simulink library "INP_IMU"  (R2024b)
settings: Solver=VariableStepAuto  StartTime=0.0  StopTime=10.0  RelTol=1e-3
libraries: INP_IMU_Comp2 x1, INP_IMU_ManOver2 x1, INP_IMU_ManOverAngRat2 x1, INP_IMU_PrepAngRat2 x1, INP_IMU_Prep2 x1
settings Model: Creator=blatak  LastModifiedBy=jmbsp
settings RTWCC: GPUComputeCapability=3.5

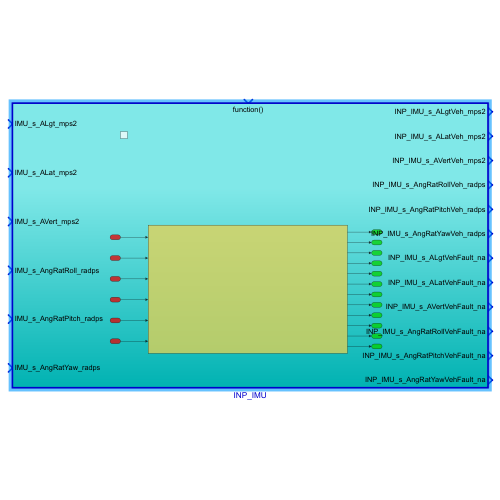
[thumbnail: Simulink's stored preview of the top-level diagram]
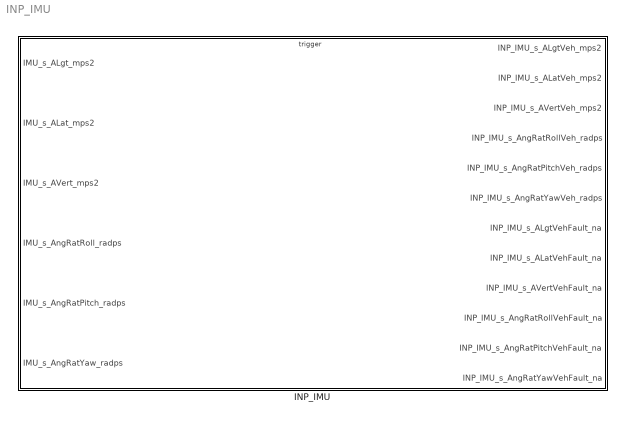
== system INP_IMU ==
  INP_IMU : Subsystem  Description=|  TreatAsAtomicUnit=on
      | Block recalculates the raw acceleration value from sensor position to cog, low
      | pass filtering, manual switches and saturation

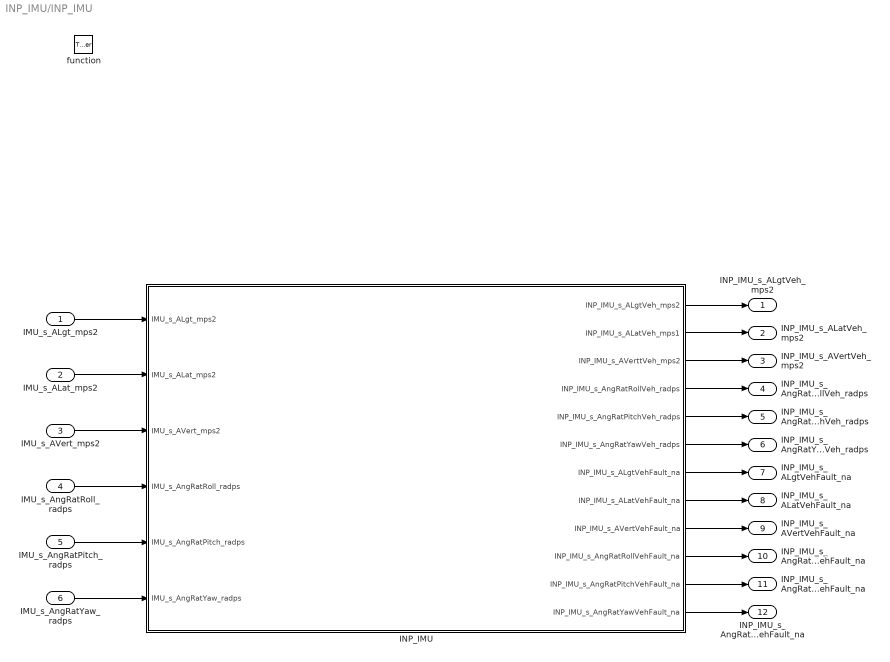
== system INP_IMU/INP_IMU ==
  IMU_s_ALgt_mps2 : Inport  Description=IMU Longitudinal acceleration - raw measured value from sensor
  IMU_s_ALat_mps2 : Inport  Description=IMU Lateral acceleration - raw measured value from sensor  Port=2
  IMU_s_AVert_mps2 : Inport  Description=IMU Vertical acceleration - raw measured value from sensor  Port=3
  IMU_s_AngRatRoll_radps : Inport  Description=IMU Angular roll velocity - raw measured value from sensor  Port=4
  IMU_s_AngRatPitch_radps : Inport  Description=IMU Angular pitch velocity - raw measured value from sensor  Port=5
  IMU_s_AngRatYaw_radps : Inport  Description=IMU Angular yaw velocity - raw measured value from sensor  Port=6
  function : TriggerPort  TriggerType=function-call  VariantControl=(inherit)
  INP_IMU : Subsystem  Description=|
      | Block recalculates the raw acceleration value from sensor position to cog, low
      | pass filtering, manual switches and saturation
  INP_IMU_s_ALgtVeh_mps2 : Outport  Description=|
      | INP IMU Longitudinal acceleration - filtered, recalculated to physical value if necessary, 
      | recalculated to cog position, saturated etc.
  INP_IMU_s_ALatVeh_mps2 : Outport  Description=|  Port=2
      | INP IMU Lateral acceleration - filtered, recalculated to physical value if necessary, 
      | recalculated to cog position, saturated etc.
  INP_IMU_s_AVertVeh_mps2 : Outport  Description=|  Port=3
      | INP IMU Vertical acceleration - filtered, recalculated to physical value if necessary, 
      | recalculated to cog position, saturated etc.
  INP_IMU_s_AngRatRollVeh_radps : Outport  Description=|  Port=4
      | INP IMU Roll velocity - filtered, recalculated to physical value if necessary,
      | saturated etc.
  INP_IMU_s_AngRatPitchVeh_radps : Outport  Description=|  Port=5
      | INP IMU Pitch velocity - filtered, recalculated to physical value if necessary,
      | saturated etc.
  INP_IMU_s_AngRatYawVeh_radps : Outport  Description=|  Port=6
      | INP IMU Yaw velocity - filtered, recalculated to physical value if necessary,
      | saturated etc.
  INP_IMU_s_ALgtVehFault_na : Outport  Port=7
  INP_IMU_s_ALatVehFault_na : Outport  Port=8
  INP_IMU_s_AVertVehFault_na : Outport  Port=9
  INP_IMU_s_AngRatRollVehFault_na : Outport  Port=10
  INP_IMU_s_AngRatPitchVehFault_na : Outport  Port=11
  INP_IMU_s_AngRatYawVehFault_na : Outport  Port=12
  wires:
  IMU_s_ALgt_mps2/1 -> INP_IMU/1(IMU_s_ALgt_mps2)
  IMU_s_ALat_mps2/1 -> INP_IMU/2(IMU_s_ALat_mps2)
  IMU_s_AVert_mps2/1 -> INP_IMU/3(IMU_s_AVert_mps2)
  IMU_s_AngRatYaw_radps/1 -> INP_IMU/6(IMU_s_AngRatYaw_radps)
  IMU_s_AngRatPitch_radps/1 -> INP_IMU/5(IMU_s_AngRatPitch_radps)
  IMU_s_AngRatRoll_radps/1 -> INP_IMU/4(IMU_s_AngRatRoll_radps)
  INP_IMU/1(INP_IMU_s_ALgtVeh_mps2) -> INP_IMU_s_ALgtVeh_mps2/1
  INP_IMU/2(INP_IMU_s_ALatVeh_mps1) -> INP_IMU_s_ALatVeh_mps2/1
  INP_IMU/3(INP_IMU_s_AVerttVeh_mps2) -> INP_IMU_s_AVertVeh_mps2/1
  INP_IMU/4(INP_IMU_s_AngRatRollVeh_radps) -> INP_IMU_s_AngRatRollVeh_radps/1
  INP_IMU/5(INP_IMU_s_AngRatPitchVeh_radps) -> INP_IMU_s_AngRatPitchVeh_radps/1
  INP_IMU/6(INP_IMU_s_AngRatYawVeh_radps) -> INP_IMU_s_AngRatYawVeh_radps/1
  INP_IMU/7(INP_IMU_s_ALgtVehFault_na) -> INP_IMU_s_ALgtVehFault_na/1
  INP_IMU/8(INP_IMU_s_ALatVehFault_na) -> INP_IMU_s_ALatVehFault_na/1
  INP_IMU/9(INP_IMU_s_AVertVehFault_na) -> INP_IMU_s_AVertVehFault_na/1
  INP_IMU/10(INP_IMU_s_AngRatRollVehFault_na) -> INP_IMU_s_AngRatRollVehFault_na/1
  INP_IMU/11(INP_IMU_s_AngRatPitchVehFault_na) -> INP_IMU_s_AngRatPitchVehFault_na/1
  INP_IMU/12(INP_IMU_s_AngRatYawVehFault_na) -> INP_IMU_s_AngRatYawVehFault_na/1

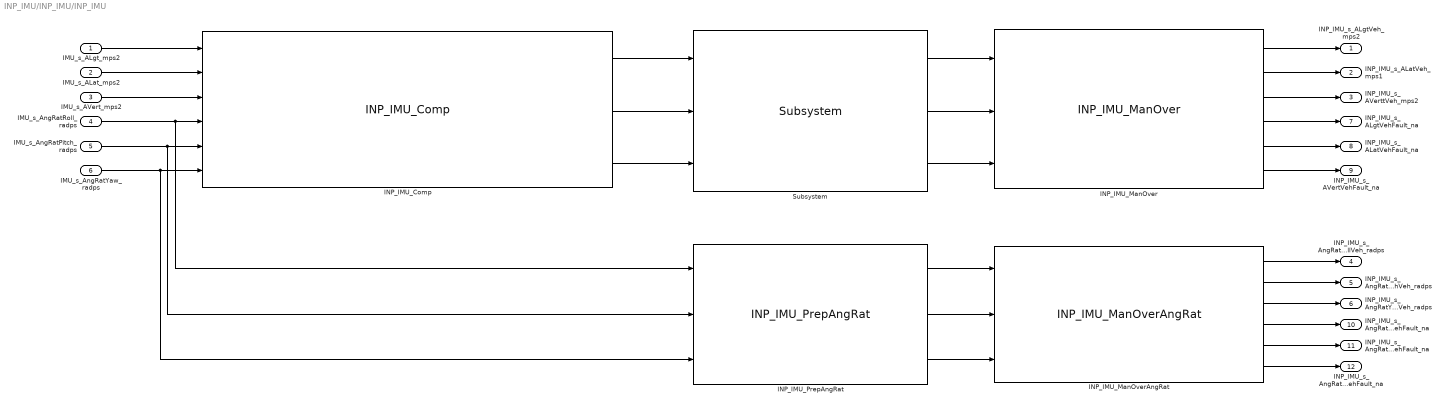
== system INP_IMU/INP_IMU/INP_IMU ==
  IMU_s_ALgt_mps2 : Inport  Description=IMU Longitudinal acceleration - raw measured value from sensor
  IMU_s_ALat_mps2 : Inport  Description=IMU Lateral acceleration - raw measured value from sensor  Port=2
  IMU_s_AVert_mps2 : Inport  Description=IMU Vertical acceleration - raw measured value from sensor  Port=3
  IMU_s_AngRatRoll_radps : Inport  Description=IMU Angular roll velocity - raw measured value from sensor  Port=4
  IMU_s_AngRatPitch_radps : Inport  Description=IMU Angular pitch velocity - raw measured value from sensor  Port=5
  IMU_s_AngRatYaw_radps : Inport  Description=IMU Angular yaw velocity - raw measured value from sensor  Port=6
  INP_IMU_Comp : INP_IMU_Comp2/INP_IMU_Comp  Description=Block compensates measured accelerations from IMU position to cog  SystemSampleTime=-1  VariantActivationTime=update diagram  AllowFlexibleInterface=on  Latency=0  AutoFrameSizeCalculation=off
  INP_IMU_ManOver : INP_IMU_ManOver2/INP_IMU_ManOver  SystemSampleTime=-1  VariantActivationTime=update diagram  AllowFlexibleInterface=on  Latency=0  AutoFrameSizeCalculation=off
  INP_IMU_ManOverAngRat : INP_IMU_ManOverAngRat2/INP_IMU_ManOverAngRat  SystemSampleTime=-1  VariantActivationTime=update diagram  AllowFlexibleInterface=on  Latency=0  AutoFrameSizeCalculation=off
  INP_IMU_PrepAngRat : INP_IMU_PrepAngRat2/INP_IMU_PrepAngRat  SystemSampleTime=-1  VariantActivationTime=update diagram  AllowFlexibleInterface=on  Latency=0  AutoFrameSizeCalculation=off
  Subsystem : INP_IMU_Prep2/Subsystem  SystemSampleTime=-1  VariantActivationTime=update diagram  AllowFlexibleInterface=on  Latency=0  AutoFrameSizeCalculation=off
  INP_IMU_s_ALgtVeh_mps2 : Outport  Description=|
      | INP IMU Longitudinal acceleration - filtered, recalculated to physical value if necessary, 
      | recalculated to cog position, saturated etc.
  INP_IMU_s_ALatVeh_mps1 : Outport  Description=|  Port=2
      | INP IMU Lateral acceleration - filtered, recalculated to physical value if necessary, 
      | recalculated to cog position, saturated etc.
  INP_IMU_s_AVerttVeh_mps2 : Outport  Description=|  Port=3
      | INP IMU Vertical acceleration - filtered, recalculated to physical value if necessary, 
      | recalculated to cog position, saturated etc.
  INP_IMU_s_AngRatRollVeh_radps : Outport  Description=|  Port=4
      | INP IMU Roll velocity - filtered, recalculated to physical value if necessary,
      | saturated etc.
  INP_IMU_s_AngRatPitchVeh_radps : Outport  Description=|  Port=5
      | INP IMU Pitch velocity - filtered, recalculated to physical value if necessary,
      | saturated etc.
  INP_IMU_s_AngRatYawVeh_radps : Outport  Description=|  Port=6
      | INP IMU Yaw velocity - filtered, recalculated to physical value if necessary,
      | saturated etc.
  INP_IMU_s_ALgtVehFault_na : Outport  Port=7
  INP_IMU_s_ALatVehFault_na : Outport  Port=8
  INP_IMU_s_AVertVehFault_na : Outport  Port=9
  INP_IMU_s_AngRatRollVehFault_na : Outport  Port=10
  INP_IMU_s_AngRatPitchVehFault_na : Outport  Port=11
  INP_IMU_s_AngRatYawVehFault_na : Outport  Port=12
  wires:
  INP_IMU_ManOverAngRat/2 -> INP_IMU_s_AngRatPitchVeh_radps/1
  IMU_s_AngRatPitch_radps/1 -> INP_IMU_PrepAngRat/2, INP_IMU_Comp/5
  INP_IMU_ManOver/1 -> INP_IMU_s_ALgtVeh_mps2/1
  INP_IMU_ManOverAngRat/3 -> INP_IMU_s_AngRatYawVeh_radps/1
  IMU_s_AngRatRoll_radps/1 -> INP_IMU_PrepAngRat/1, INP_IMU_Comp/4
  INP_IMU_ManOver/3 -> INP_IMU_s_AVerttVeh_mps2/1
  Subsystem/2 -> INP_IMU_ManOver/2
  INP_IMU_Comp/1 -> Subsystem/1
  INP_IMU_PrepAngRat/2 -> INP_IMU_ManOverAngRat/2
  INP_IMU_PrepAngRat/3 -> INP_IMU_ManOverAngRat/3
  INP_IMU_PrepAngRat/1 -> INP_IMU_ManOverAngRat/1
  INP_IMU_ManOverAngRat/1 -> INP_IMU_s_AngRatRollVeh_radps/1
  IMU_s_ALgt_mps2/1 -> INP_IMU_Comp/1
  INP_IMU_Comp/3 -> Subsystem/3
  IMU_s_AngRatYaw_radps/1 -> INP_IMU_PrepAngRat/3, INP_IMU_Comp/6
  IMU_s_ALat_mps2/1 -> INP_IMU_Comp/2
  INP_IMU_ManOver/2 -> INP_IMU_s_ALatVeh_mps1/1
  IMU_s_AVert_mps2/1 -> INP_IMU_Comp/3
  INP_IMU_Comp/2 -> Subsystem/2
  Subsystem/1 -> INP_IMU_ManOver/1
  Subsystem/3 -> INP_IMU_ManOver/3
  INP_IMU_ManOver/4 -> INP_IMU_s_ALgtVehFault_na/1
  INP_IMU_ManOver/5 -> INP_IMU_s_ALatVehFault_na/1
  INP_IMU_ManOver/6 -> INP_IMU_s_AVertVehFault_na/1
  INP_IMU_ManOverAngRat/4 -> INP_IMU_s_AngRatRollVehFault_na/1
  INP_IMU_ManOverAngRat/5 -> INP_IMU_s_AngRatPitchVehFault_na/1
  INP_IMU_ManOverAngRat/6 -> INP_IMU_s_AngRatYawVehFault_na/1
